simulink model "q01"  (R2024a)
settings: Solver=FixedStepAuto  StartTime=0.0  StopTime=65  FixedStep=1  RelTol=1e-3
settings Model: Creator=amir  LastModifiedBy=amir

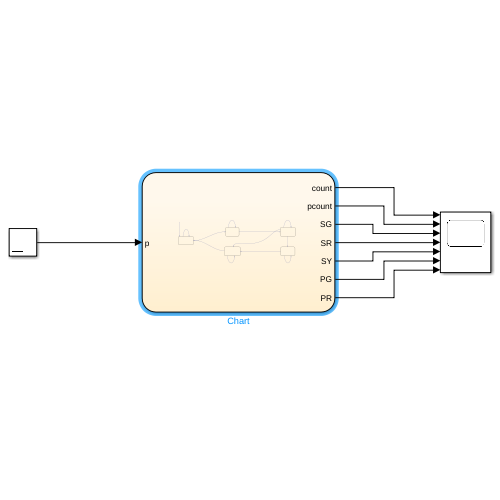
[thumbnail: Simulink's stored preview of the top-level diagram]
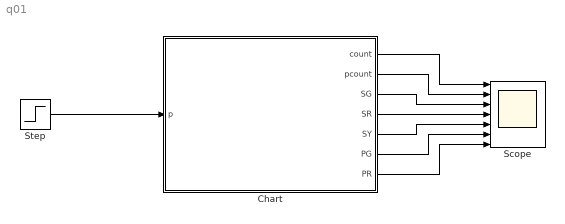
== system q01 ==
  Chart : Stateflow chart  TreatAsAtomicUnit=on
  Scope : Scope  NumInputPorts=7
  Step : Step  SampleTime=0
  wires:
  Chart/1(count) -> Scope/1
  Chart/2(pcount) -> Scope/2
  Step/1 -> Chart/1(p)
  Chart/3(SG) -> Scope/3
  Chart/4(SR) -> Scope/4
  Chart/5(SY) -> Scope/5
  Chart/6(PG) -> Scope/6
  Chart/7(PR) -> Scope/7

== stateflow chart q01/Chart ==
  state carred_pedred
  state cargreen_pedred
  state carred_pedgreen
  state caryellow_pedred
  state pending_pedred
  cargreen_pedred -> cargreen_pedred [order 1] : [count<60]{count=count+1; SG=0;}
  carred_pedred -> carred_pedred [order 2] : /{count=count+1; PR=0;}
  (default) -> carred_pedgreen : {count=0; pcount=0}
  carred_pedgreen -> carred_pedgreen [order 2] : {count=count+1; pcount=pcount+1; SR=0; PG=0;}
  cargreen_pedred -> caryellow_pedred [order 3] : [p && count>=60]{count=0; SY=1;}
  carred_pedgreen -> carred_pedred [order 1] : [pcount>=55]{count=count+1; PR=1;}
  carred_pedred -> cargreen_pedred [order 1] : [count>=60]{count=count+1; SG=1; PR=0;}
  cargreen_pedred -> pending_pedred [order 2] : [p==1 && count<60]{SG=0;}
  caryellow_pedred -> carred_pedgreen [order 1] : [pcount>=5]{count=0; pcount=0; SR=1; PG=1; SG=0; SY=0;}
  pending_pedred -> caryellow_pedred [order 1] : [pcount>=60]{count=0; SY=1}
  caryellow_pedred -> caryellow_pedred [order 2] : {count=count+1; SY=0;}
  pending_pedred -> pending_pedred [order 2] : {count=count+1}
  data: p input; count output; pcount output; SG output; SR output; SY output; PG output; PR output
